simulink model "Klimaanlage"  (R2023b)
settings: Solver=FixedStepAuto  StartTime=0.0  StopTime=1000  RelTol=1e-3  EnableMultiTasking=on
values from neighbouring files (symbols this model uses):
  T_a = 5    [integration_test_01.m]
  T_i_start = 10    [integration_test_01.m]
libraries: mbedblockslib x10, nucleoboard_ac_controll_software x1, thermical_vehicelbody x1
settings Model: ExtModeTrigDuration=10  Creator=kilia  LastModifiedBy=kilia
settings OptimizationCC: UseDivisionForNetSlopeComputation=on  GainParamInheritBuiltInType=on  UseFloatMulNetSlope=on  PassReuseOutputArgsThreshold=0  EfficientFloat2IntCast=on  MaxStackSize=64  OptimizeBlockOrder=speed  DifferentSizesBufferReuse=on
settings DebuggingCC: ParameterTunabilityLossMsg=error
settings HardwareCC: ProdBitPerPointer=32  ProdBitPerSizeT=32  ProdBitPerPtrDiffT=32  ProdLargestAtomicInteger=Long  ProdLargestAtomicFloat=Double  ProdWordSize=32  ProdLongLongMode=on  ProdHWDeviceType=ARM Compatible->ARM Cortex  TargetBitPerPointer=64  TargetBitPerSizeT=64  TargetBitPerPtrDiffT=64  TargetLongLongMode=on  TargetIntDivRoundTo=Zero  TargetEndianess=LittleEndian  TargetWordSize=64  TargetHWDeviceType=MATLAB Host  ProdEqTarget=off
settings SFSimCC: MATLABDynamicMemAlloc=off
settings RTWCC: Description=S-Function Target  SystemTargetFile=rtwsfcn.tlc  TemplateMakefile=rtwsfcn_default_tmf  Toolchain=GNU Tools for ARM Embedded Processors
settings CodeAppCC: ForceParamTrailComments=on  OperatorAnnotations=on
settings STFCustomTargetCC: TargetLangStandard=C89/C90 (ANSI)  ModelReferenceCompliant=off  CompOptLevelCompliant=on  MATLABClassNameForMDSCustomization=Simulink.SoftwareTarget.TargetSpecificTriggerConfigurationBase  GRTInterface=on  SystemTargetFile=rtwsfcn.tlc

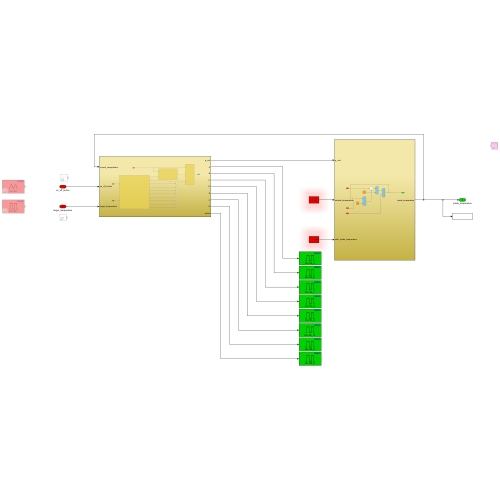
[thumbnail: Simulink's stored preview of the top-level diagram]
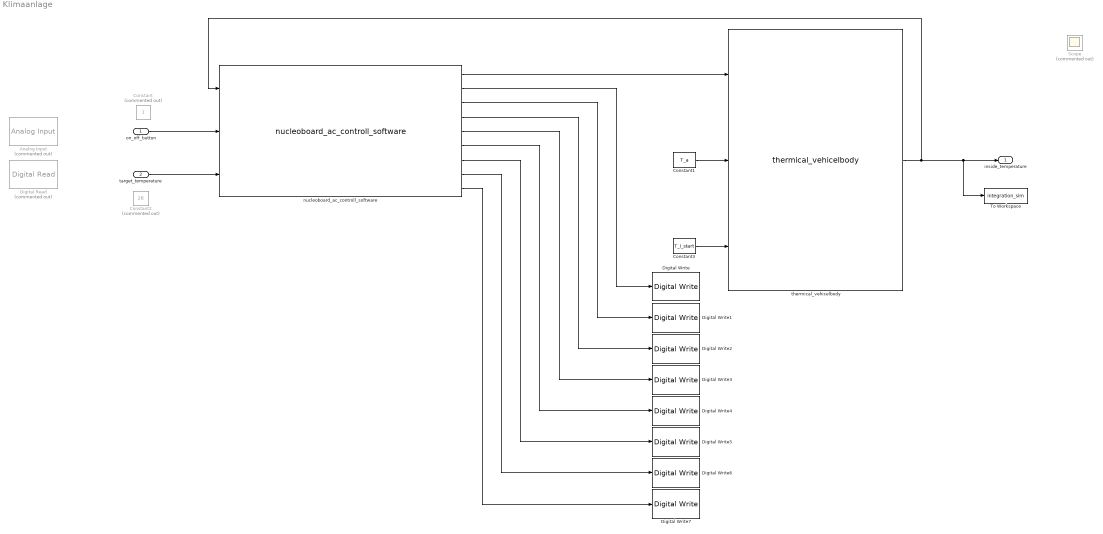
== system Klimaanlage ==
  on_off_button : Inport  OutDataTypeStr=boolean
  target_temperature : Inport  Port=2
  Analog Input : mbedblockslib/Analog Input  Commented=on  Pin=A0  ReadResultsOnly=off  ConversionTriggerSource=Software  ExternalTriggerType=uint32( 0 )  OutputDataType=double  EnableConversionCompleteNotify=off  EnableOuputStatus=off  SampleTime=-1
      settings: LibrarySourceBlock=stmnucleorootlib/Common/Analog Input
  Constant : Constant  Commented=on  OutDataTypeStr=boolean
  Constant1 : Constant  Value=T_a
  Constant2 : Constant  Commented=on  Value=28  OutDataTypeStr=uint16
  Constant3 : Constant  Value=T_i_start
  Digital Read : mbedblockslib/Digital Read  Commented=on  Pin=D2  Direction=input  SampleTime=-1
      settings: LibrarySourceBlock=stmnucleorootlib/Common/Digital Read
  Digital Write : mbedblockslib/Digital Write  Pin=PA_5  Direction=output
      settings: LibrarySourceBlock=stmnucleorootlib/Common/Digital Write
  Digital Write1 : mbedblockslib/Digital Write  Pin=PA_6  Direction=output
      settings: LibrarySourceBlock=stmnucleorootlib/Common/Digital Write
  Digital Write2 : mbedblockslib/Digital Write  Pin=PA_7  Direction=output
      settings: LibrarySourceBlock=stmnucleorootlib/Common/Digital Write
  Digital Write3 : mbedblockslib/Digital Write  Pin=PA_8  Direction=output
      settings: LibrarySourceBlock=stmnucleorootlib/Common/Digital Write
  Digital Write4 : mbedblockslib/Digital Write  Pin=PA_9  Direction=output
      settings: LibrarySourceBlock=stmnucleorootlib/Common/Digital Write
  Digital Write5 : mbedblockslib/Digital Write  Pin=PA_15  Direction=output
      settings: LibrarySourceBlock=stmnucleorootlib/Common/Digital Write
  Digital Write6 : mbedblockslib/Digital Write  Pin=PB_9  Direction=output
      settings: LibrarySourceBlock=stmnucleorootlib/Common/Digital Write
  Digital Write7 : mbedblockslib/Digital Write  Pin=PB_0  Direction=output
      settings: LibrarySourceBlock=stmnucleorootlib/Common/Digital Write
  Scope : Scope  Commented=on
  To Workspace : ToWorkspace  VariableName=integration_sim  SaveFormat=Timeseries  SampleTime=-1
  nucleoboard_ac_controll_software : nucleoboard_ac_controll_software/nucleoboard_ac_controll_software  SystemSampleTime=-1  VariantActivationTime=update diagram  AllowFlexibleInterface=on  Latency=0  AutoFrameSizeCalculation=off
  thermical_vehicelbody : thermical_vehicelbody/thermical_vehicelbody  SystemSampleTime=-1  VariantActivationTime=update diagram  AllowFlexibleInterface=on  Latency=0  AutoFrameSizeCalculation=off
  inside_temperature : Outport
  wires:
  Constant1/1 -> thermical_vehicelbody/2
  nucleoboard_ac_controll_software/1 -> thermical_vehicelbody/1
  Constant3/1 -> thermical_vehicelbody/3
  target_temperature/1 -> nucleoboard_ac_controll_software/3
  on_off_button/1 -> nucleoboard_ac_controll_software/2
  thermical_vehicelbody/1 -> To Workspace/1, inside_temperature/1, nucleoboard_ac_controll_software/1
  nucleoboard_ac_controll_software/2 -> Digital Write/1
  nucleoboard_ac_controll_software/3 -> Digital Write1/1
  nucleoboard_ac_controll_software/4 -> Digital Write2/1
  nucleoboard_ac_controll_software/5 -> Digital Write3/1
  nucleoboard_ac_controll_software/6 -> Digital Write4/1
  nucleoboard_ac_controll_software/7 -> Digital Write5/1
  nucleoboard_ac_controll_software/8 -> Digital Write6/1
  nucleoboard_ac_controll_software/9 -> Digital Write7/1
